simulink model "Model_1"  (R2016b)
settings: Solver=ode23s  StartTime=0.0  StopTime=1  RelTol=1e-3
InitFcn:
  | init
values from neighbouring files (symbols this model uses):
  Kctrl = 1e-6    (= 1e-06)    [SharifNejad.m]
settings Model: Creator=Mojtaba  LastModifiedBy=Mojtaba

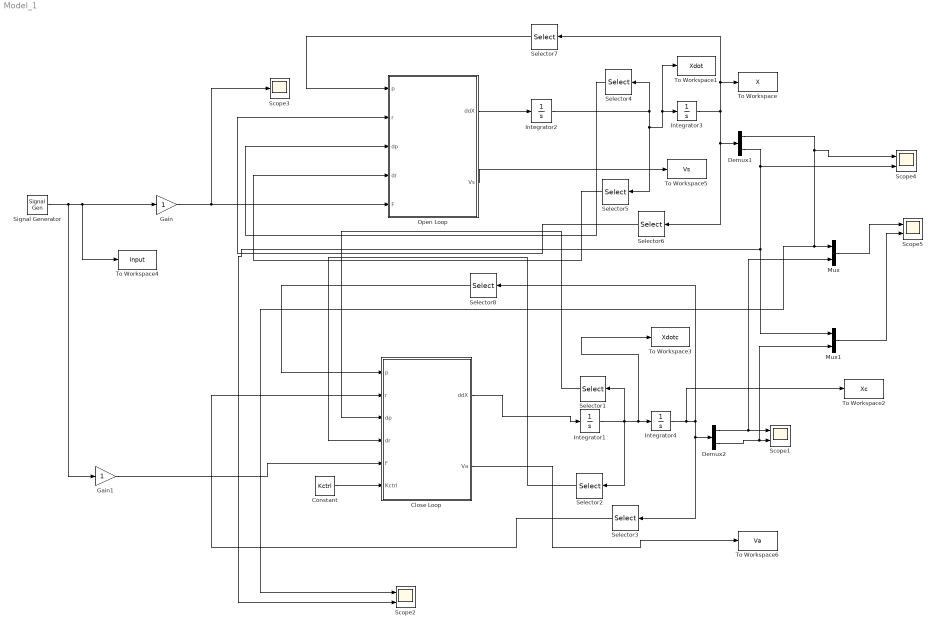
== system Model_1 ==
  Close Loop : MATLAB Function  TreatAsAtomicUnit=on
  Constant : Constant  Value=Kctrl
  Demux1 : Demux  Outputs=2
  Demux2 : Demux  Outputs=2
  Gain : Gain
  Gain1 : Gain
  Integrator{1..4} (4 alike) : Integrator  InitialCondition=[0;0]
  Mux : Mux  Inputs=2
  Mux1 : Mux  Inputs=2
  Open Loop : MATLAB Function  TreatAsAtomicUnit=on
  Scope{1..2,4..5} (4 alike) : Scope  NumInputPorts=2
  Scope3 : Scope
  Selector{1,4,7..8} (4 alike) : Selector  InputPortWidth=2  IndexOptions=Index vector (dialog)  Indices=[1]  OutputSizes=1
  Selector{2..3,5..6} (4 alike) : Selector  InputPortWidth=2  IndexOptions=Index vector (dialog)  Indices=[2]  OutputSizes=1
  Signal Generator : SignalGenerator  WaveForm=square  Amplitude=10  Frequency=10
  To Workspace : ToWorkspace  VariableName=X  SaveFormat=Structure With Time  SampleTime=-1
  To Workspace1 : ToWorkspace  VariableName=Xdot  SaveFormat=Structure With Time  SampleTime=-1
  To Workspace2 : ToWorkspace  VariableName=Xc  SaveFormat=Structure With Time  SampleTime=-1
  To Workspace3 : ToWorkspace  VariableName=Xdotc  SaveFormat=Structure With Time  SampleTime=-1
  To Workspace4 : ToWorkspace  VariableName=Input  SaveFormat=Structure With Time  SampleTime=-1
  To Workspace5 : ToWorkspace  VariableName=Vs  SaveFormat=Structure With Time  SampleTime=-1
  To Workspace6 : ToWorkspace  VariableName=Va  SaveFormat=Structure With Time  SampleTime=-1
  wires:
  Open Loop/1(ddX) -> Integrator2/1
  Integrator2/1 -> Selector5/1, To Workspace1/1, Integrator3/1, Selector4/1
  Integrator3/1 -> Demux1/1, Selector6/1, To Workspace/1, Selector7/1
  Selector5/1 -> Open Loop/4(dr)
  Selector4/1 -> Open Loop/3(dp)
  Selector6/1 -> Open Loop/2(r)
  Selector7/1 -> Open Loop/1(p)
  Demux1/2 -> Scope4/2, Mux1/1, Scope2/2
  Gain/1 -> Scope3/1, Open Loop/5(F)
  Close Loop/1(ddX) -> Integrator1/1
  Integrator1/1 -> Selector1/1, To Workspace3/1, Integrator4/1, Selector2/1
  Integrator4/1 -> To Workspace2/1, Selector8/1, Selector3/1, Demux2/1
  Signal Generator/1 -> Gain/1, To Workspace4/1, Gain1/1
  Selector2/1 -> Close Loop/4(dr)
  Selector1/1 -> Close Loop/3(dp)
  Selector3/1 -> Close Loop/2(r)
  Selector8/1 -> Close Loop/1(p)
  Demux2/1 -> Mux/2, Scope1/1
  Demux2/2 -> Mux1/2, Scope1/2
  Gain1/1 -> Close Loop/5(F)
  Mux/1 -> Scope5/1
  Mux1/1 -> Scope5/2
  Open Loop/2(Vs) -> To Workspace5/1
  Close Loop/2(Va) -> To Workspace6/1
  Demux1/1 -> Scope4/1, Scope2/1, Mux/1
  Constant/1 -> Close Loop/6(Kctrl)

== matlab function Model_1/Open Loop ==
  data: p input; ddX output; r input; dp input; dr input; F input; Vs output
function [ddX,Vs] = fcn(p,r,dp,dr,F)
M=[0.01,0;0,.46756];
K=[.121e9,-.0378e9;-.0378e9,4.37596e9];
Q=[0;1.444];
Cp=zeros(2);
C1=[-3.7268e8,-1.7284e8];
X=[p;r];
dX=[dp;dr];
F=F.*eye(2);
ddX=pinv(M)*((F*Q)-(K*X)-(Cp*dX));
Vs=C1*X;

== matlab function Model_1/Close Loop ==
  data: p input; ddX output; r input; dp input; dr input; F input; Va output; Kctrl input
function [ddX,Va] = fcn(p,r,dp,dr,F,Kctrl)
% global Kctrl
% K=system.K;
% Q=system.Q;
% Cp=system.Cp;
% global M K Q 
%#codegen
M=[0.01,0;0,.46756];
K=[.121e9,-.0378e9;-.0378e9,4.37596e9];
Q=[0;1.444];


% Cp=1.*[3.67348e18,-9.9523e18;3.67348e18,-9.95227e18];
% Cp=[5.41687,-2.487;2.5122,-1.153].*1e2;
% Gain=[3.7268,1.7284].*1e3;
X=[p;r];
dX=[dp;dr];
F=[F,0;0,F];
Cp=[5.416877014077774  -2.487500077826886
    2.512210343500663  -1.153639524902399].*1e7;
Cp=Kctrl.*Cp;
ddX=pinv(M)*((F*Q)-(K*X)-(Cp*dX));
C1=[-3.7268,-1.7284].*1e8;
Gain=-Kctrl*C1';
Gain=Gain';
Va=Gain*dX;
end
